simulink model "lab4simulinktask12"  (Simulink 7.7)
settings: Solver=ode45  StartTime=0.0  StopTime=10.0  RelTol=1e-3
libraries: cstblocks x3
settings Model: Creator=Muhammad Ali khan  LastModifiedBy=Muhammad Ali khan

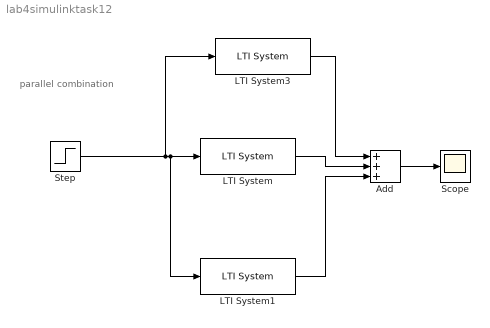
== system lab4simulinktask12 ==
  note: parallel combination
  Add : Sum  Inputs=+++
  LTI System : cstblocks/LTI System  SystemSampleTime=-1  sys=tf([1 ],[1 1])  IC=[]
  LTI System1 : cstblocks/LTI System  SystemSampleTime=-1  sys=tf([1],[1 3])  IC=[]
  LTI System3 : cstblocks/LTI System  SystemSampleTime=-1  sys=tf([1 ],[1 1])  IC=[]
  Scope : Scope
  Step : Step  SampleTime=0
  wires:
  Step/1 -> LTI System3/1, LTI System/1, LTI System1/1
  LTI System/1 -> Add/2
  LTI System3/1 -> Add/1
  LTI System1/1 -> Add/3
  Add/1 -> Scope/1
